simulink model "model_sim_2023"  (R2023b)
settings: Solver=VariableStepAuto  StartTime=0.0  StopTime=10  MaxStep=1e-3  RelTol=1e-3
values from neighbouring files (symbols this model uses):
  a = double(py.config.a)    [simulation__data.m]    (also in speed_to_PWM.m)
  a_log = double(py.config.a_log)    [simulation__data.m]
  b = double(py.config.b)    [simulation__data.m]    (also in speed_to_PWM.m)
  b_log = double(py.config.b_log)    [simulation__data.m]
  c = double(py.config.c)    [simulation__data.m]    (also in speed_to_PWM.m)
  d = real(d)*sy + sqrt(-1)*imag(d)*sx    [nyquist1.m]    (also in simulation__data.m = double(py.config.d); speed_to_PWM.m = double(py.config.d))
  Kp = double(py.config.Kp)    [simulation__data.m]
  max_PWM = double(py.config.MAX_PWM)    [simulation__data.m]
  max_speed = double(py.config.MAX_SPEED)    [simulation__data.m]
  pulse_zero = pulse_min    (= 10)    [simulation__data.m]
  step_0_pulse_1 = 0    [simulation__data.m]
  step_value = 20    [simulation__data.m]
  x0 = 50    [simulation__data.m]
settings Model: Creator=feder  LastModifiedBy=federico-romairone
settings RTWCC: GPUComputeCapability=5.0
settings ConfigComp: CovBoundaryAbsTol=1.0e-5

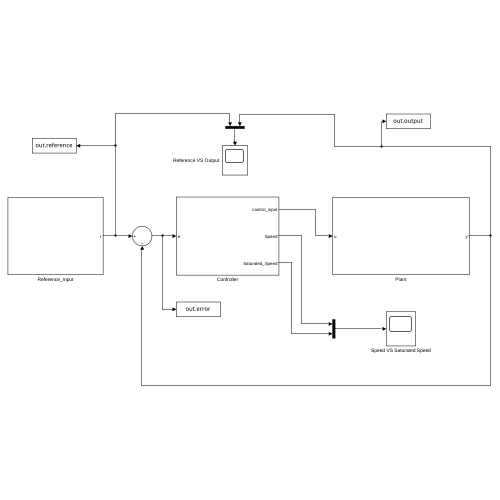
[thumbnail: Simulink's stored preview of the top-level diagram]
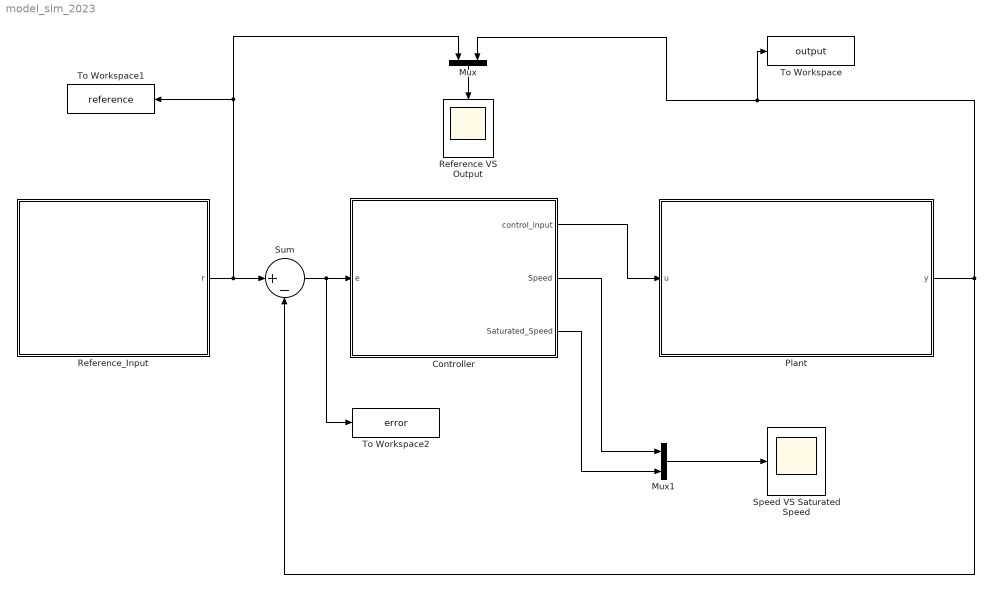
== system model_sim_2023 ==
  Controller : Subsystem
  Mux : Mux  Inputs=2
  Mux1 : Mux  Inputs=2
  Plant : Subsystem
  Reference VS Output : Scope
  Reference_Input : Subsystem
  Speed VS Saturated Speed : Scope
  Sum : Sum  Inputs=|+-
  To Workspace : ToWorkspace  VariableName=output  SaveFormat=Timeseries  SampleTime=-1
  To Workspace1 : ToWorkspace  VariableName=reference  SaveFormat=Timeseries  SampleTime=-1
  To Workspace2 : ToWorkspace  VariableName=error  SaveFormat=Timeseries  SampleTime=-1
  wires:
  Plant/1(y) -> Mux/2, To Workspace/1, Sum/2
  Sum/1 -> To Workspace2/1, Controller/1(e)
  Controller/1(control_input) -> Plant/1(u)
  Mux/1 -> Reference VS Output/1
  Mux1/1 -> Speed VS Saturated Speed/1
  Controller/2(Speed) -> Mux1/1
  Controller/3(Saturated_Speed) -> Mux1/2
  Reference_Input/1(r) -> To Workspace1/1, Mux/1, Sum/1

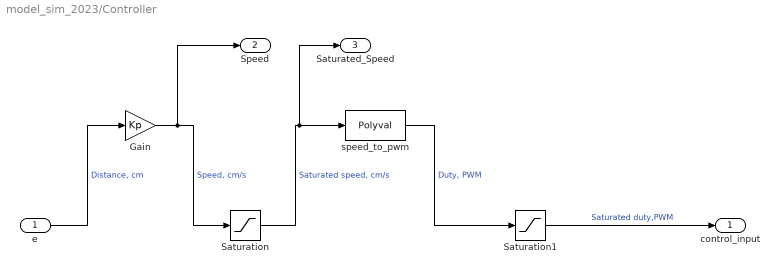
== system model_sim_2023/Controller ==
  e : Inport
  Gain : Gain  Gain=Kp
  Saturation : Saturate  UpperLimit=max_speed  LowerLimit=-max_speed
  Saturation1 : Saturate  UpperLimit=max_PWM  LowerLimit=-max_PWM
  speed_to_pwm : Polyval  Coefs=[ a, b, c, d ]
  control_input : Outport
  Speed : Outport  Port=2
  Saturated_Speed : Outport  Port=3
  wires:
  e/1 -> Gain/1  "Distance, cm"
  Gain/1 -> Speed/1, Saturation/1  "Speed, cm/s"
  Saturation/1 -> speed_to_pwm/1, Saturated_Speed/1  "Saturated speed, cm/s"
  speed_to_pwm/1 -> Saturation1/1  "Duty, PWM"
  Saturation1/1 -> control_input/1  "Saturated duty,PWM"

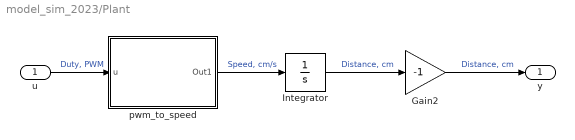
== system model_sim_2023/Plant ==
  u : Inport
  Gain2 : Gain  Gain=-1
  Integrator : Integrator  InitialCondition=-x0
  pwm_to_speed : Subsystem
  y : Outport
  wires:
  Integrator/1 -> Gain2/1  "Distance, cm"
  pwm_to_speed/1(Out1) -> Integrator/1  "Speed, cm/s"
  Gain2/1 -> y/1  "Distance, cm"
  u/1 -> pwm_to_speed/1(u)  "Duty, PWM"

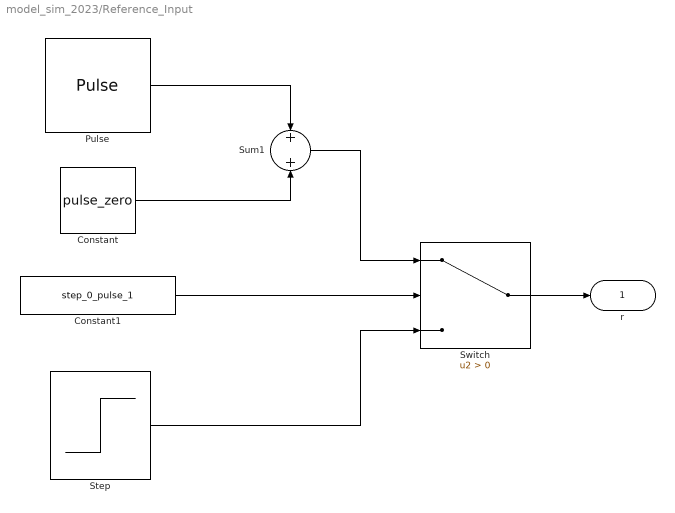
== system model_sim_2023/Reference_Input ==
  Constant : Constant  Value=pulse_zero
  Constant1 : Constant  Value=step_0_pulse_1
  Pulse : DiscretePulseGenerator  PulseType=Time based  Amplitude=10  Period=4  PulseWidth=50
  Step : Step  Time=0  After=step_value  SampleTime=0
  Sum1 : Sum
  Switch : Switch  Criteria=u2 > Threshold  SaturateOnIntegerOverflow=off  InputSameDT=off
  r : Outport
  wires:
  Pulse/1 -> Sum1/1
  Constant/1 -> Sum1/2
  Constant1/1 -> Switch/2
  Sum1/1 -> Switch/1
  Step/1 -> Switch/3
  Switch/1 -> r/1

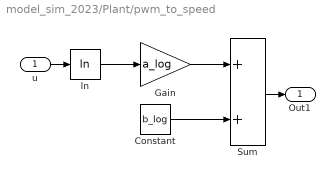
== system model_sim_2023/Plant/pwm_to_speed ==
  u : Inport
  Constant : Constant  Value=b_log
  Gain : Gain  Gain=a_log
  Sum : Sum
  ln : Math  Operator=log
  Out1 : Outport
  wires:
  Gain/1 -> Sum/1
  ln/1 -> Gain/1
  Constant/1 -> Sum/2
  Sum/1 -> Out1/1
  u/1 -> ln/1
